simulink model "ideal_switch_inverter_one_ph_x3"  (R2025a)
settings: Solver=daessc  StartTime=0.0  StopTime=0.2  MaxStep=1e-7  RelTol=1e-3
undefined symbols (not defined in the file): Down, Up
libraries: ee_lib x33, fl_lib x19, nesl_utility x17, eePwmGenerator x6, spsMeanLib x3, simulink x2, spsRMSLib x1
settings Model: SimulationMode=rapid-accelerator  Creator=alexey  LastModifiedBy=alexey
settings SolverCC: ZeroCrossAlgorithm=Adaptive
settings OptimizationCC: ReuseModelBlockBuffer=off
settings DebuggingCC: IgnoredZcDiagnostic=none
settings RTWCC: GPUComputeCapability=3.5
settings GRTTargetCC: RTWCAPISignals=on  RTWCAPIParams=on

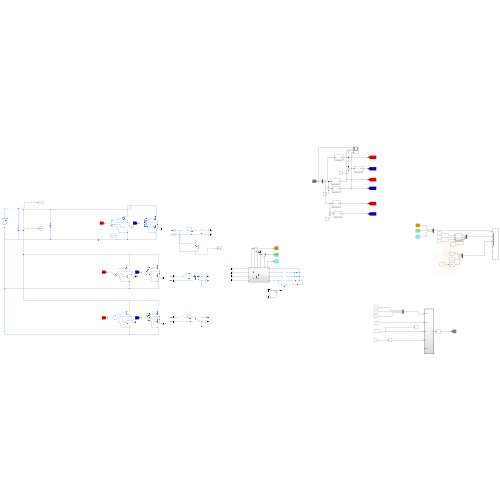
[thumbnail: Simulink's stored preview of the top-level diagram]
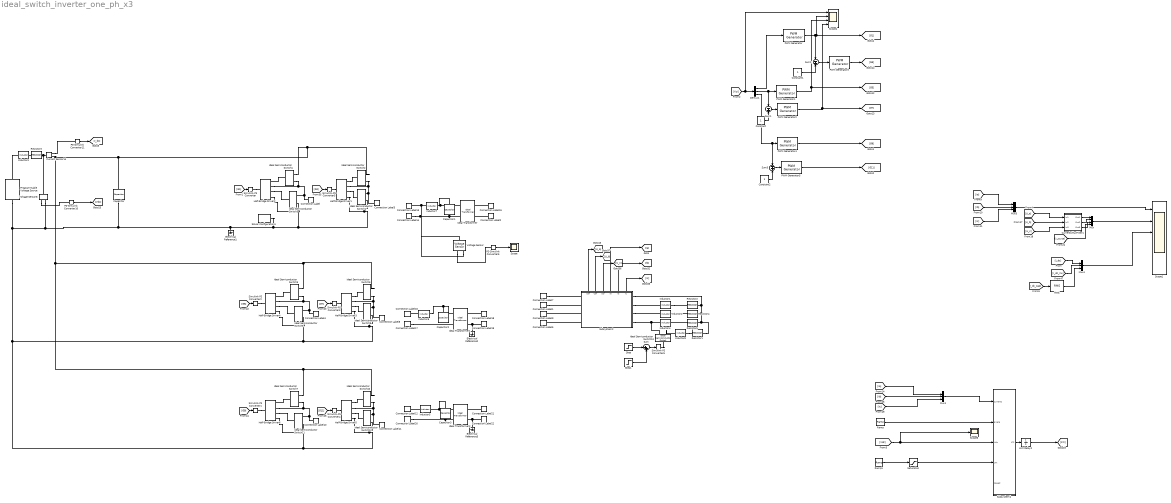
== system ideal_switch_inverter_one_ph_x3 ==
  Capacitor : fl_lib/Electrical/Electrical Elements/Capacitor  c=900 uF  r=1e-6 Ohm  g=0 1/Ohm  i_specify=off  i_priority=None  i=0 A  i_nominal_specify=off  i_nominal_value=1  i_nominal_unit=A  v_specify=off  v_priority=None  v=0 V  v_nominal_specify=off  v_nominal_value=1  v_nominal_unit=V  vc_specify=off  vc_priority=High  vc=0 V  vc_nominal_specify=off  vc_nominal_value=1  vc_nominal_unit=V
  Capacitor1 : fl_lib/Electrical/Electrical Elements/Capacitor  c=100 uF  r=2 mOhm  g=0 1/Ohm  i_specify=off  i_priority=None  i=0 A  i_nominal_specify=off  i_nominal_value=1  i_nominal_unit=A  v_specify=on  v_priority=None  v=0 V  v_nominal_specify=off  v_nominal_value=1  v_nominal_unit=V  vc_specify=off  vc_priority=High  vc=0 V  vc_nominal_specify=off  vc_nominal_value=1  vc_nominal_unit=V
  Capacitor2 : fl_lib/Electrical/Electrical Elements/Capacitor  c=100 uF  r=2 mOhm  g=0 1/Ohm  i_specify=off  i_priority=None  i=0 A  i_nominal_specify=off  i_nominal_value=1  i_nominal_unit=A  v_specify=on  v_priority=None  v=0 V  v_nominal_specify=off  v_nominal_value=1  v_nominal_unit=V  vc_specify=off  vc_priority=High  vc=0 V  vc_nominal_specify=off  vc_nominal_value=1  vc_nominal_unit=V
  Capacitor3 : fl_lib/Electrical/Electrical Elements/Capacitor  c=100 uF  r=2 mOhm  g=0 1/Ohm  i_specify=off  i_priority=None  i=0 A  i_nominal_specify=off  i_nominal_value=1  i_nominal_unit=A  v_specify=on  v_priority=None  v=0 V  v_nominal_specify=off  v_nominal_value=1  v_nominal_unit=V  vc_specify=off  vc_priority=High  vc=0 V  vc_nominal_specify=off  vc_nominal_value=1  vc_nominal_unit=V
  Connection Label : ConnectionLabel  Label=A01
  Connection Label1 : ConnectionLabel  Label=A
  Connection Label10 : ConnectionLabel  Label=C01
  Connection Label11 : ConnectionLabel  Label=C02
  Connection Label12 : ConnectionLabel  Label=C01
  Connection Label13 : ConnectionLabel  Label=A01
  Connection Label14 : ConnectionLabel  Label=A02
  Connection Label15 : ConnectionLabel  Label=A
  Connection Label16 : ConnectionLabel  Label=B01
  Connection Label17 : ConnectionLabel  Label=B02
  Connection Label18 : ConnectionLabel  Label=B
  Connection Label{2,7,19,22} (4 alike) : ConnectionLabel  Label=N
  Connection Label20 : ConnectionLabel  Label=C02
  Connection Label21 : ConnectionLabel  Label=C
  Connection Label3 : ConnectionLabel  Label=A02
  Connection Label4 : ConnectionLabel  Label=B01
  Connection Label5 : ConnectionLabel  Label=C
  Connection Label8 : ConnectionLabel  Label=B02
  Connection Label9 : ConnectionLabel  Label=B
  Constant : Constant
  Constant1 : Constant
  Constant2 : Constant
  Current Sensor14 : fl_lib/Electrical/Electrical Sensors/Current Sensor
  CurrentsMuxFilter1 : Subsystem
  Demux1 : Demux  Outputs=3
  Electrical Reference1 : fl_lib/Electrical/Electrical Elements/Electrical Reference
  Electrical Reference2 : fl_lib/Electrical/Electrical Elements/Electrical Reference
  Electrical Reference3 : fl_lib/Electrical/Electrical Elements/Electrical Reference
  Half-Bridge Driver{1..6} (6 alike) : ee_lib/Semiconductors & Converters/Half-Bridge Driver  port_option=ee.enum.controlport.ps  uHigh=2.0 V  uLow=0.8 V  uHighValue=0.7  uLowValue=0.3  vHigh=15 V  vLow=0 V  tpLH=50 ns  tdLH=1 ns  tpHL=50 ns  tdHL=1 ns  parameterization=ee.enum.semiconductors.gateDriverParam.outputImpedance  rHigh=2 Ohm  rLow=2 Ohm  tRise=20 ns  tFall=20 ns  cLoad=10 nF  ZonTime_specify=off  ZonTime_priority=None  ZonTime=0 s  ZoffTime_specify=off  ZoffTime_priority=None  ZoffTime=0 s  power_dissipated_high_side_specify=off  power_dissipated_high_side_priority=None  power_dissipated_high_side=0 W  power_dissipated_high_side_nominal_specify=off  power_dissipated_high_side_nominal_value=1  power_dissipated_high_side_nominal_unit=W  power_dissipated_low_side_specify=off  power_dissipated_low_side_priority=None  power_dissipated_low_side=0 W  power_dissipated_low_side_nominal_specify=off  power_dissipated_low_side_nominal_value=1  power_dissipated_low_side_nominal_unit=W
      settings: InternalSimscapePortConfiguration="{\"Bottom\":[],\"Left\":[{\"id\":\"u\",\"label\":\"u\",\"type\":\"input\"}],\"Right\":[{\"id\":\"HO\",\"label\":\"HO\",\"type\":\"foundation.electrical.electrical\"},{\"id\":\"HS\",\"label\":\"HS\",\"type\":\"foundation.electrical.electrical\"},{\"id\":\"LO\",\"label\":\"LO\",\"type\":\"foundation.electrical.electrical\"},{\"id\":\"LS\",\"label\":\"LS\",\"type\":\"foundation.electrical.electrical\"}],\"Top\":[]}"
  Ideal Semiconductor Switch{1..12} (12 alike) : ee_lib/Semiconductors & Converters/Ideal Semiconductor Switch  port_option=ee.enum.controlport.elec  Ron=0.001 Ohm  Goff=1e-6 1/Ohm  Vth=10 V  diode_param=ee.enum.semiconductors.protectionDiode.nodynamics  diode_Vf=0.8 V  diode_Ron=0.001 Ohm  diode_Goff=1e-5 1/Ohm  diode_C=50e-9 F  diode_iRM=-235 A  diode_iF=300 A  diode_idot=-50 A/us  diode_trr_param=ee.enum.converters.diodetrr.trr_factor  diode_trr_factor=3  diode_trr=15 us  diode_Qrr=1500 s*uA
      settings: InternalSimscapePortConfiguration="{\"Bottom\":[],\"Left\":[{\"id\":\"G_elec\",\"label\":\"\",\"type\":\"foundation.electrical.electrical\"}],\"Right\":[{\"id\":\"A\",\"label\":\"a\",\"type\":\"foundation.electrical.electrical\"},{\"id\":\"K\",\"label\":\"k\",\"type\":\"foundation.electrical.electrical\"}],\"Top\":[]}"
  Ideal Semiconductor Switch13 : ee_lib/Semiconductors & Converters/Ideal Semiconductor Switch  port_option=ee.enum.controlport.ps  Ron=0.001 Ohm  Goff=1e-6 1/Ohm  Vth=1.5 V  diode_param=ee.enum.semiconductors.protectionDiode.external  diode_Vf=0.8 V  diode_Ron=0.001 Ohm  diode_Goff=1e-5 1/Ohm  diode_C=50e-9 F  diode_iRM=-235 A  diode_iF=300 A  diode_idot=-50 A/us  diode_trr_param=ee.enum.converters.diodetrr.trr_factor  diode_trr_factor=3  diode_trr=15 us  diode_Qrr=1500 s*uA
  Ideal Transformer : fl_lib/Electrical/Electrical Elements/Ideal Transformer  n=1  i1_specify=off  i1_priority=None  i1=0 A  i1_nominal_specify=off  i1_nominal_value=1  i1_nominal_unit=A  v1_specify=off  v1_priority=None  v1=0 V  v1_nominal_specify=off  v1_nominal_value=1  v1_nominal_unit=V  i2_specify=off  i2_priority=None  i2=0 A  i2_nominal_specify=off  i2_nominal_value=1  i2_nominal_unit=A  v2_specify=off  v2_priority=None  v2=0 V  v2_nominal_specify=off  v2_nominal_value=1  v2_nominal_unit=V
  Ideal Transformer1 : fl_lib/Electrical/Electrical Elements/Ideal Transformer  n=1  i1_specify=off  i1_priority=None  i1=0 A  i1_nominal_specify=off  i1_nominal_value=1  i1_nominal_unit=A  v1_specify=off  v1_priority=None  v1=0 V  v1_nominal_specify=off  v1_nominal_value=1  v1_nominal_unit=V  i2_specify=off  i2_priority=None  i2=0 A  i2_nominal_specify=off  i2_nominal_value=1  i2_nominal_unit=A  v2_specify=off  v2_priority=None  v2=0 V  v2_nominal_specify=off  v2_nominal_value=1  v2_nominal_unit=V
  Ideal Transformer2 : fl_lib/Electrical/Electrical Elements/Ideal Transformer  n=1  i1_specify=off  i1_priority=None  i1=0 A  i1_nominal_specify=off  i1_nominal_value=1  i1_nominal_unit=A  v1_specify=off  v1_priority=None  v1=0 V  v1_nominal_specify=off  v1_nominal_value=1  v1_nominal_unit=V  i2_specify=off  i2_priority=None  i2=0 A  i2_nominal_specify=off  i2_nominal_value=1  i2_nominal_unit=A  v2_specify=off  v2_priority=None  v2=0 V  v2_nominal_specify=off  v2_nominal_value=1  v2_nominal_unit=V
  Inductor{1..2,4,8} (4 alike) : ee_lib/Passive/Inductor  l=3630 uH  enable_L_tol=0  L_tol=20  tol_distribution=1  nSigma=4  r=0 Ohm  g=1e-9 1/Ohm  enable_operating_limits=0  operating_limit_action=2  max_working_current=1 A  power_rating=1 W  i_L_specify=on  i_L_priority=High  i_L=0 A  i_L_nominal_specify=off  i_L_nominal_value=1  i_L_nominal_unit=A
  Inductor3 : ee_lib/Passive/Inductor  l=1 uH  enable_L_tol=0  L_tol=20  tol_distribution=1  nSigma=4  r=0 Ohm  g=1e-9 1/Ohm  enable_operating_limits=0  operating_limit_action=2  max_working_current=1 A  power_rating=1 W  i_L_specify=on  i_L_priority=High  i_L=0 A  i_L_nominal_specify=off  i_L_nominal_value=1  i_L_nominal_unit=A
  Inductor5 : ee_lib/Passive/Inductor  l=200 uH  enable_L_tol=0  L_tol=20  tol_distribution=1  nSigma=4  r=0 Ohm  g=1e-9 1/Ohm  enable_operating_limits=0  operating_limit_action=2  max_working_current=1 A  power_rating=1 W  i_L_specify=on  i_L_priority=High  i_L=0 A  i_L_nominal_specify=off  i_L_nominal_value=1  i_L_nominal_unit=A
  Inductor6 : ee_lib/Passive/Inductor  l=200 uH  enable_L_tol=0  L_tol=20  tol_distribution=1  nSigma=4  r=0 Ohm  g=1e-9 1/Ohm  enable_operating_limits=0  operating_limit_action=2  max_working_current=1 A  power_rating=1 W  i_L_specify=on  i_L_priority=High  i_L=0 A  i_L_nominal_specify=off  i_L_nominal_value=1  i_L_nominal_unit=A
  Inductor7 : ee_lib/Passive/Inductor  l=200 uH  enable_L_tol=0  L_tol=20  tol_distribution=1  nSigma=4  r=0 Ohm  g=1e-9 1/Ohm  enable_operating_limits=0  operating_limit_action=2  max_working_current=1 A  power_rating=1 W  i_L_specify=on  i_L_priority=High  i_L=0 A  i_L_nominal_specify=off  i_L_nominal_value=1  i_L_nominal_unit=A
  Mux : Mux
  Mux1 : Mux  Inputs=3
  Mux3 : Mux  Inputs=3
  Mux4 : Mux  Inputs=3
  PS-Simulink Converter10 : nesl_utility/PS-Simulink Converter  PhysicalDomain=network_engine_domain  SubClassName=ps_output  LeftPortType=input  RightPortType=output  PseudoPeriodic=off  Frequencies=[]  VectorFormat=inherit  Unit=inherit  AffineConversion=off
  PS-Simulink Converter11 : nesl_utility/PS-Simulink Converter  PhysicalDomain=network_engine_domain  SubClassName=ps_output  LeftPortType=input  RightPortType=output  PseudoPeriodic=off  Frequencies=[]  VectorFormat=inherit  Unit=inherit  AffineConversion=off
  PS-Simulink Converter5 : nesl_utility/PS-Simulink Converter  PhysicalDomain=network_engine_domain  SubClassName=ps_output  LeftPortType=input  RightPortType=output  PseudoPeriodic=off  Frequencies=[]  VectorFormat=inherit  Unit=inherit  AffineConversion=off
  PWM Generator{,1..5} (6 alike) : eePwmGenerator/PWM Generator  CarrCount=Up-Down  Tper=0.5/10000  Tdelay=0  Ts=100e-9
  Programmable Voltage Source : ee_lib/Sources/Programmable Voltage Source  magnitude_type=ee.enum.timechanging.constant  ac_magnitude=0 V  magn_ramp=1 V/s  magn_step=1 V  magn_modu_magn=1 V  magn_modu_freq=1 Hz  magn_t1=1 s  magn_t2=2 s  frequency_type=ee.enum.timechanging.constant  ac_frequency=60 Hz  freq_ramp=1 Hz/s  freq_step=1 Hz  freq_modu_magn=1 Hz  freq_modu_freq=1 Hz  freq_t1=1 s  freq_t2=2 s  phase_type=ee.enum.timechanging.constant  ac_shift=0 deg  phase_ramp=1 deg/s  phase_step=1 deg  phase_modu_magn=1 deg  phase_modu_freq=1 Hz  phase_t1=1 s  phase_t2=2 s  dc_type=ee.enum.timechanging.ramp  dc_voltage=0 V  dc_ramp=450000 V/s  dc_step=24 V  dc_modu_magn=1 V  dc_modu_freq=1 Hz  dc_t1=0 s  dc_t2=100e-5 s  harmonic_option=0  harmonic_orders=[5, 7, 11, 13]  harmonic_ratios=[.1, .1, .1, .1]  harmonic_shifts=[0, 0, 0, 0] deg  harmonic_t1=-inf s  harmonic_t2=inf s  noise_mode=0  PSD=0 V^2/Hz  repeatability=1  auto_seed=0  user_seed=0  sample_time=1e-3 s  i_specify=off  i_priority=None  i=0 A  i_nominal_specify=off  i_nominal_value=1  i_nominal_unit=A  v_specify=on  v_priority=High  v=0 V  v_nominal_specify=off  v_nominal_value=1  v_nominal_unit=V
      settings: InternalSimscapePortConfiguration="{\"Bottom\":[],\"Left\":[{\"id\":\"p\",\"label\":\"+\",\"type\":\"foundation.electrical.electrical\"}],\"Right\":[{\"id\":\"n\",\"label\":\"-\",\"type\":\"foundation.electrical.electrical\"}],\"Top\":[]}"
  RMS : spsRMSLib/RMS  TrueRMS=on  Freq=1000  RMSInit=0  Ts=0
  Ramp : simulink/Sources/Ramp  slope=100*pi  start=0  InitialOutput=0
  Ramp1 : simulink/Sources/Ramp  slope=7500  start=0  InitialOutput=0
  Resistor1 : ee_lib/Passive/Resistor  R=1.52 Ohm  enable_R_tol=0  R_tol=5  tol_distribution=1  nSigma=4  enable_operating_limits=0  operating_limit_action=2  power_rating=1 W  max_working_voltage=100 V  noise_mode=0  Tdevice=25 degC  sample_time=1e-3 s  repeatability=1  user_seed=0  auto_seed=1003532619  power_derating_T1=70 degC  power_derating_T2=155 degC  operating_temperature_range_vec=[-50, 150] degC  alpha=3.93e-3 1/K  Tmeas=25 degC  thermal_mass=100 J/K  temperature_specify=off  temperature_priority=High  temperature=298.15 K  temperature_nominal_specify=off  temperature_nominal_value=1  temperature_nominal_unit=K
  Resistor2 : ee_lib/Passive/Resistor  R=1.52 Ohm  enable_R_tol=0  R_tol=5  tol_distribution=1  nSigma=4  enable_operating_limits=0  operating_limit_action=2  power_rating=1 W  max_working_voltage=100 V  noise_mode=0  Tdevice=25 degC  sample_time=1e-3 s  repeatability=1  user_seed=0  auto_seed=1045931777  power_derating_T1=70 degC  power_derating_T2=155 degC  operating_temperature_range_vec=[-50, 150] degC  alpha=3.93e-3 1/K  Tmeas=25 degC  thermal_mass=100 J/K  temperature_specify=off  temperature_priority=High  temperature=298.15 K  temperature_nominal_specify=off  temperature_nominal_value=1  temperature_nominal_unit=K
  Resistor3 : ee_lib/Passive/Resistor  R=1 mOhm  enable_R_tol=0  R_tol=5  tol_distribution=1  nSigma=4  enable_operating_limits=0  operating_limit_action=2  power_rating=1 W  max_working_voltage=100 V  noise_mode=0  Tdevice=25 degC  sample_time=1e-3 s  repeatability=1  user_seed=0  auto_seed=545404223  power_derating_T1=70 degC  power_derating_T2=155 degC  operating_temperature_range_vec=[-50, 150] degC  alpha=3.93e-3 1/K  Tmeas=25 degC  thermal_mass=100 J/K  temperature_specify=off  temperature_priority=High  temperature=298.15 K  temperature_nominal_specify=off  temperature_nominal_value=1  temperature_nominal_unit=K
  Resistor4 : ee_lib/Passive/Resistor  R=1.52 Ohm  enable_R_tol=0  R_tol=5  tol_distribution=1  nSigma=4  enable_operating_limits=0  operating_limit_action=2  power_rating=1 W  max_working_voltage=100 V  noise_mode=0  Tdevice=25 degC  sample_time=1e-3 s  repeatability=1  user_seed=0  auto_seed=844370171  power_derating_T1=70 degC  power_derating_T2=155 degC  operating_temperature_range_vec=[-50, 150] degC  alpha=3.93e-3 1/K  Tmeas=25 degC  thermal_mass=100 J/K  temperature_specify=off  temperature_priority=High  temperature=298.15 K  temperature_nominal_specify=off  temperature_nominal_value=1  temperature_nominal_unit=K
  Resistor5 : ee_lib/Passive/Resistor  R=1.52 Ohm  enable_R_tol=0  R_tol=5  tol_distribution=1  nSigma=4  enable_operating_limits=0  operating_limit_action=2  power_rating=1 W  max_working_voltage=100 V  noise_mode=0  Tdevice=25 degC  sample_time=1e-3 s  repeatability=1  user_seed=0  auto_seed=1078396959  power_derating_T1=70 degC  power_derating_T2=155 degC  operating_temperature_range_vec=[-50, 150] degC  alpha=3.93e-3 1/K  Tmeas=25 degC  thermal_mass=100 J/K  temperature_specify=off  temperature_priority=High  temperature=298.15 K  temperature_nominal_specify=off  temperature_nominal_value=1  temperature_nominal_unit=K
  Saturation : Saturate  UpperLimit=450
  Scope : Scope
      settings: ActiveDisplayYMinimum=-551.33280842234649  ActiveDisplayYMaximum=616.82988904528236
  Scope1 : Scope  NumInputPorts=6
      settings: ActiveDisplayString=6  ActiveDisplayYMinimum=-1  ActiveDisplayYMaximum=1
  Scope4 : Scope  NumInputPorts=4
      settings: ActiveDisplayYMinimum=-0.081880277547520586  ActiveDisplayYMaximum=0.73692249792768538  DataLoggingVariableName=ScopeData2
  Scope6 : Scope
      settings: ActiveDisplayYMinimum=-58.427844353684108  ActiveDisplayYMaximum=525.8505991831571  DataLoggingVariableName=ScopeData4
  Simulink-PS Converter{,1..6} (7 alike) : nesl_utility/Simulink-PS Converter  PhysicalDomain=network_engine_domain  SubClassName=ps_input  LeftPortType=input  RightPortType=output  PseudoPeriodic=off  Frequencies=[]  NoiseDistribution=none  NoiseParameters=[]  Unit=1  AffineConversion=off  FilteringAndDerivatives=provide  SimscapeFilterOrder=1  InputFilterTimeConstant=0.001  UdotUserProvided=0
  Solver Configuration1 : nesl_utility/Solver Configuration  PhysicalDomain=network_engine_domain  SubClassName=solver  LeftPortType=input  RightPortType=generic  Tones=[]  Harmonics=[]  SimulateNoise=off  Profile=off  UseLocalSampling=off  EnableSwitchedLinearOptims=on  FrequencyDomain=off  UseCCode=off  RelTol=0.001  AbsTol=0.001  MinStep=1e-09  ToWorkspace=off  RevertToSquareIcSolve=off  NumHomotopyIterations=100  PhasorMode=off  PhasorModeNumHarmonics=1  ConsistencySolver=NEWTON_XTOL_AFTER_FTOL  IndexReductionMethod=DerivativeReplacement  DoDC=off  ResidualTolerance=1e-09  ConsistencyTolSource=GLOBAL  ConsistencyAbsTol=0.001  ConsistencyRelTol=0.001  ConsistencyTolFactor=0.001  UseLocalSolver=off  LocalSolverChoice=NE_BACKWARD_EULER_ADVANCER  ResolveIndetEquations=on  FunctionEvalNumThread=1  LocalSolverSampleTime=0.001  DoFixedCost=off  MaxNonlinIter=3  MaxModeIter=2  ComputeImpulses=off  ImpulseIterations=2  LinearAlgebra=auto  LinearAlgebraNumThread=0  EquationFormulation=NE_TIME_EF  DelaysMemoryBudget=1024  AutomaticFiltering=on  FilteringTimeConstant=0.001  PartitionStorageMethod=AS_NEEDED  PartitionMemoryBudget=1024  PartitionMethod=ROBUST  MultibodyUseLocalSolver=off  MultibodyLocalSolverChoice=ODE1  MultibodyLocalSolverSampleTime=0.001
  Step : Step  Time=0.08  SampleTime=0
  Step1 : Step  Time=0.12  Before=1  After=0  SampleTime=0
  Subsystem1 : Subsystem  TreatAsAtomicUnit=on  SystemSampleTime=1/10000
  Subsystem2 : Subsystem
      settings: PortSchema="{\"entries\":[{\"content\":{\"sides\":[{\"content\":{},\"type\":\"ConnectorPlacement.EquallySpacedRectSide\",\"uuid\":\"18ff9a98-da5f-4d42-bf88-8b80acaefaab\"},{\"content\":{\"connectorIds\":[\"Out1\",\"Out2\",\"Out3\",\"Out4\",\"Out5\",\"Out6\"],\"side\":\"RIGHT\"},\"type\":\"ConnectorPlacement.EquallySpacedRectSide\",\"uuid\":\"2ae2e449-c022-4e43-8d74-e7903f555369\"},{\"content\":{\"connectorIds\":[\"LConn1\",\"LConn2\",\"LConn3\",\"LConn4\"],\"side\":\"TOP\"},\"type\":\"ConnectorPlacement.EquallySpacedRectSide\",\"uuid\":\"55b123c9-903d-428f-ba92-02a5913ccae5\"},{\"content\":{\"connectorIds\":[\"RConn1\",\"RConn2\",\"RConn3\",\"RConn4\"],\"side\":\"BOTTOM\"},\"type\":\"ConnectorPlacement.EquallySpacedRectSide\",\"uuid\":\"b028b0af-4fd3-4535-8d3b-f50dc0cabb29\"}]},\"type\":\"ConnectorPlacement.EquallySpacedConnector\",\"uuid\":\"08d0fd08-360e-4301-974e-a78b2c2bf0b9\"}],\"packageUris\":[\"http://schema.mathworks.com/mf0/Connector/R2020b\"],\"version\":\"1.0\"}"
  Sum : Sum  Inputs=|++
  Sum1 : Sum  Inputs=-+
  Sum2 : Sum  Inputs=-+
  Sum3 : Sum  Inputs=-+
  Unit Delay2 : UnitDelay  SampleTime=-1  HasFrameUpgradeWarning=on
  Voltage Sensor : fl_lib/Electrical/Electrical Sensors/Voltage Sensor
  Voltage Sensor8 : fl_lib/Electrical/Electrical Sensors/Voltage Sensor
  wires:
  [Ib] -> Mux1/2
  [Ia] -> Mux1/1
  PS-Simulink Converter10/1 -> [Vdc]
  [G1] -> Simulink-PS Converter/1
  PS-Simulink Converter11/1 -> [I_dc]
  [G3] -> Simulink-PS Converter5/1
  [Vdc] -> Scope6/1, Subsystem1/3(Vdc)
  [I_dc] -> Mux4/1
  Subsystem1/1(KZI) -> Unit Delay2/1
  Unit Delay2/1 -> [Kzi]
  [Kzi] -> Scope4/1, Demux1/1
  Demux1/1 -> PWM Generator/1
  Demux1/2 -> PWM Generator1/1, Sum1/1
  PWM Generator1/1 -> Scope4/3, [G5]
  PWM Generator2/1 -> [G7], Scope4/4
  [I_dc_inv] -> Mux4/2
  [Ia] -> Mux3/1
  [Ib] -> Mux3/2
  [Ic] -> Mux3/3
  Mux4/1 -> Scope1/3
  Subsystem2/1(Uaf) -> [U_a]
  Subsystem2/2(Ubf) -> [U_b]
  Subsystem2/3(Ucf) -> [U_c]
  Subsystem2/4(Ia) -> [Ia]
  Subsystem2/5(Ib) -> [Ib]
  Subsystem2/6(Ic) -> [Ic]
  [U_a] -> CurrentsMuxFilter1/1(In1)
  [U_b] -> CurrentsMuxFilter1/2(In2)
  [U_c] -> CurrentsMuxFilter1/3(In3)
  CurrentsMuxFilter1/1(Out1) -> Mux/1
  CurrentsMuxFilter1/2(Out2) -> Mux/2
  CurrentsMuxFilter1/3(Out3) -> Mux/3
  Mux/1 -> Scope1/2
  Mux3/1 -> Scope1/1
  [Ic] -> Mux1/3
  Mux1/1 -> Subsystem1/1(currents)
  [v_source] -> Mux/4
  [I_dc_cap] -> RMS/1
  Ramp/1 -> Subsystem1/2(angle)
  RMS/1 -> Mux4/3
  Ramp1/1 -> Saturation/1
  Saturation/1 -> Subsystem1/4(Um)
  Constant/1 -> Sum1/2
  Sum1/1 -> PWM Generator2/1
  Sum2/1 -> PWM Generator3/1
  Constant1/1 -> Sum2/2
  PWM Generator/1 -> Scope4/2, [G1], Sum2/1
  PWM Generator3/1 -> [G3]
  [G7] -> Simulink-PS Converter3/1
  [G5] -> Simulink-PS Converter2/1
  [G9] -> Simulink-PS Converter1/1
  [G11] -> Simulink-PS Converter4/1
  Sum3/1 -> PWM Generator5/1
  Constant2/1 -> Sum3/2
  PWM Generator5/1 -> [G11]
  Demux1/3 -> Sum3/1, PWM Generator4/1
  PWM Generator4/1 -> [G9]
  Step/1 -> Sum/1
  Step1/1 -> Sum/2
  PS-Simulink Converter5/1 -> Scope/1
  Sum/1 -> Simulink-PS Converter6/1
  connections:
  Resistor3/RConn1 -- Inductor3/RConn1
  Ideal Semiconductor Switch1/LConn1 -- Half-Bridge Driver2/RConn1
  Inductor3/LConn1 -- Programmable Voltage Source/LConn1
  Half-Bridge Driver1/RConn1 -- Ideal Semiconductor Switch2/LConn1
  Current Sensor14/LConn1 -- Voltage Sensor8/LConn1 -- Resistor3/LConn1
  Half-Bridge Driver2/RConn3 -- Ideal Semiconductor Switch3/LConn1
  Voltage Sensor8/RConn1 -- PS-Simulink Converter10/LConn1
  Simulink-PS Converter5/RConn1 -- Half-Bridge Driver1/LConn1
  Simulink-PS Converter/RConn1 -- Half-Bridge Driver2/LConn1
  Current Sensor14/RConn1 -- PS-Simulink Converter11/LConn1
  Half-Bridge Driver1/RConn3 -- Ideal Semiconductor Switch4/LConn1
  Half-Bridge Driver6/RConn4 -- Half-Bridge Driver1/RConn4 -- Ideal Semiconductor Switch4/RConn2 -- Half-Bridge Driver2/RConn4 -- Ideal Semiconductor Switch3/RConn2 -- Solver Configuration1/RConn1 -- Electrical Reference1/LConn1 -- Capacitor/RConn1 -- Voltage Sensor8/RConn2 -- Programmable Voltage Source/RConn1 -- Half-Bridge Driver4/RConn4 -- Ideal Semiconductor Switch8/RConn2 -- Ideal Semiconductor Switch9/RConn2 -- Half-Bridge Driver3/RConn4 -- Half-Bridge Driver5/RConn4 -- Ideal Semiconductor Switch12/RConn2 -- Ideal Semiconductor Switch11/RConn2
  Half-Bridge Driver1/RConn2 -- Connection Label3/LConn1 -- Ideal Semiconductor Switch4/RConn1 -- Ideal Semiconductor Switch2/RConn2
  Half-Bridge Driver2/RConn2 -- Ideal Semiconductor Switch1/RConn2 -- Connection Label/LConn1 -- Ideal Semiconductor Switch3/RConn1
  Connection Label1/LConn1 -- Subsystem2/LConn3
  Subsystem2/LConn2 -- Connection Label9/LConn1
  Subsystem2/LConn1 -- Connection Label5/LConn1
  Inductor1/RConn1 -- Resistor2/RConn1
  Resistor4/RConn1 -- Inductor2/RConn1
  Resistor5/RConn1 -- Inductor4/RConn1
  Resistor2/LConn1 -- Subsystem2/RConn4 -- Resistor1/LConn1 -- Resistor5/LConn1 -- Resistor4/LConn1
  Subsystem2/RConn3 -- Inductor1/LConn1
  Subsystem2/RConn2 -- Inductor2/LConn1
  Subsystem2/RConn1 -- Inductor4/LConn1 -- Ideal Semiconductor Switch13/RConn1
  Connection Label7/LConn1 -- Subsystem2/LConn4
  Connection Label14/LConn1 -- Voltage Sensor/RConn2 -- Capacitor1/RConn1 -- Ideal Transformer/LConn2
  Ideal Transformer/LConn1 -- Capacitor1/LConn1 -- Inductor7/RConn1
  Connection Label2/LConn1 -- Ideal Transformer/RConn2
  Connection Label15/LConn1 -- Ideal Transformer/RConn1
  Connection Label17/LConn1 -- Ideal Transformer1/LConn2
  Inductor6/RConn1 -- Capacitor2/LConn1 -- Ideal Transformer1/LConn1
  Connection Label18/LConn1 -- Ideal Transformer1/RConn1
  Connection Label19/LConn1 -- Electrical Reference2/LConn1 -- Ideal Transformer1/RConn2
  Half-Bridge Driver3/RConn2 -- Ideal Semiconductor Switch6/RConn2 -- Ideal Semiconductor Switch9/RConn1 -- Connection Label8/LConn1
  Half-Bridge Driver4/RConn2 -- Ideal Semiconductor Switch8/RConn1 -- Connection Label4/LConn1 -- Ideal Semiconductor Switch5/RConn2
  Ideal Semiconductor Switch7/RConn1 -- Ideal Semiconductor Switch5/RConn1 -- Ideal Semiconductor Switch6/RConn1 -- Current Sensor14/RConn2 -- Capacitor/LConn1 -- Ideal Semiconductor Switch1/RConn1 -- Ideal Semiconductor Switch2/RConn1 -- Ideal Semiconductor Switch10/RConn1
  Half-Bridge Driver3/RConn3 -- Ideal Semiconductor Switch9/LConn1
  Simulink-PS Converter2/RConn1 -- Half-Bridge Driver4/LConn1
  Simulink-PS Converter3/RConn1 -- Half-Bridge Driver3/LConn1
  Half-Bridge Driver4/RConn3 -- Ideal Semiconductor Switch8/LConn1
  Half-Bridge Driver3/RConn1 -- Ideal Semiconductor Switch6/LConn1
  Ideal Semiconductor Switch5/LConn1 -- Half-Bridge Driver4/RConn1
  Inductor7/LConn1 -- Voltage Sensor/LConn1 -- Connection Label13/LConn1
  Inductor6/LConn1 -- Connection Label16/LConn1
  Ideal Semiconductor Switch12/RConn1 -- Half-Bridge Driver5/RConn2 -- Ideal Semiconductor Switch10/RConn2 -- Connection Label11/LConn1
  Ideal Semiconductor Switch11/RConn1 -- Half-Bridge Driver6/RConn2 -- Ideal Semiconductor Switch7/RConn2 -- Connection Label10/LConn1
  Simulink-PS Converter1/RConn1 -- Half-Bridge Driver6/LConn1
  Ideal Semiconductor Switch7/LConn1 -- Half-Bridge Driver6/RConn1
  Half-Bridge Driver5/RConn1 -- Ideal Semiconductor Switch10/LConn1
  Half-Bridge Driver5/RConn3 -- Ideal Semiconductor Switch12/LConn1
  Simulink-PS Converter4/RConn1 -- Half-Bridge Driver5/LConn1
  Half-Bridge Driver6/RConn3 -- Ideal Semiconductor Switch11/LConn1
  Connection Label20/LConn1 -- Capacitor3/RConn1 -- Ideal Transformer2/LConn2
  Ideal Transformer2/LConn1 -- Capacitor3/LConn1 -- Inductor5/RConn1
  Electrical Reference3/LConn1 -- Connection Label22/LConn1 -- Ideal Transformer2/RConn2
  Connection Label21/LConn1 -- Ideal Transformer2/RConn1
  Inductor5/LConn1 -- Connection Label12/LConn1
  Voltage Sensor/RConn1 -- PS-Simulink Converter5/LConn1
  Simulink-PS Converter6/RConn1 -- Ideal Semiconductor Switch13/LConn1
  Inductor8/RConn1 -- Resistor1/RConn1
  Ideal Semiconductor Switch13/RConn2 -- Inductor8/LConn1

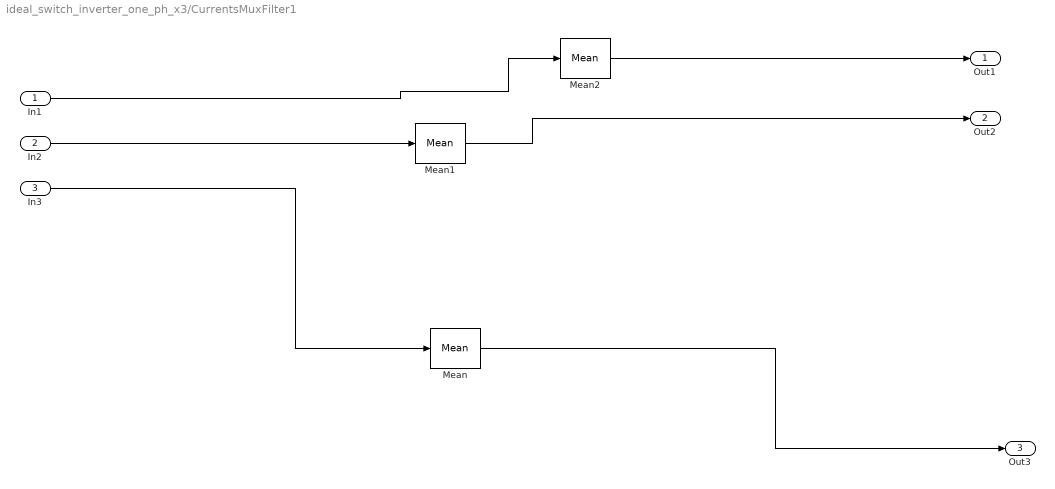
== system ideal_switch_inverter_one_ph_x3/CurrentsMuxFilter1 ==
  In1 : Inport
  In2 : Inport  Port=2
  In3 : Inport  Port=3
  Mean : spsMeanLib/Mean  Freq=10000  Vinit=0  Ts=0
  Mean1 : spsMeanLib/Mean  Freq=10000  Vinit=0  Ts=0
  Mean2 : spsMeanLib/Mean  Freq=10000  Vinit=0  Ts=0
  Out1 : Outport
  Out2 : Outport  Port=2
  Out3 : Outport  Port=3
  wires:
  In1/1 -> Mean2/1
  In3/1 -> Mean/1
  In2/1 -> Mean1/1
  Mean/1 -> Out3/1
  Mean1/1 -> Out2/1
  Mean2/1 -> Out1/1

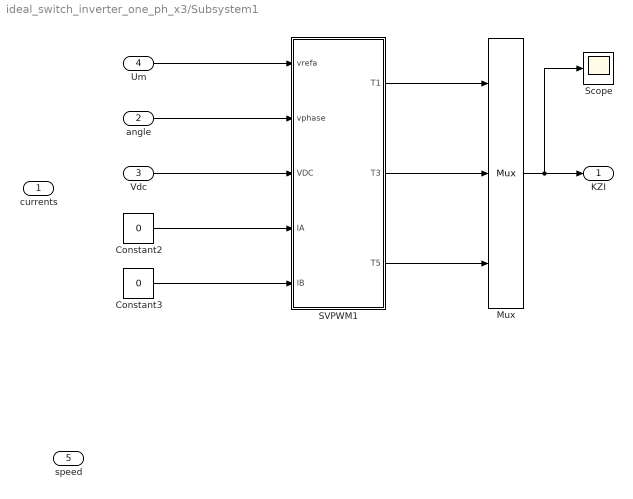
== system ideal_switch_inverter_one_ph_x3/Subsystem1 ==
  currents : Inport
  angle : Inport  Port=2
  Vdc : Inport  Port=3
  Um : Inport  Port=4
  speed : Inport  Port=5
  Constant2 : Constant  Value=0
  Constant3 : Constant  Value=0
  Mux : Mux  Inputs=3
  SVPWM1 : MATLAB Function  TreatAsAtomicUnit=on
  Scope : Scope
      settings: ActiveDisplayYMinimum=0.18750000000000003  ActiveDisplayYMaximum=0.8125  DataLoggingVariableName=ScopeData3
  KZI : Outport
  wires:
  SVPWM1/1(T1) -> Mux/1
  SVPWM1/2(T3) -> Mux/2
  SVPWM1/3(T5) -> Mux/3
  Mux/1 -> Scope/1, KZI/1
  Um/1 -> SVPWM1/1(vrefa)
  Vdc/1 -> SVPWM1/3(VDC)
  angle/1 -> SVPWM1/2(vphase)
  Constant2/1 -> SVPWM1/4(IA)
  Constant3/1 -> SVPWM1/5(IB)

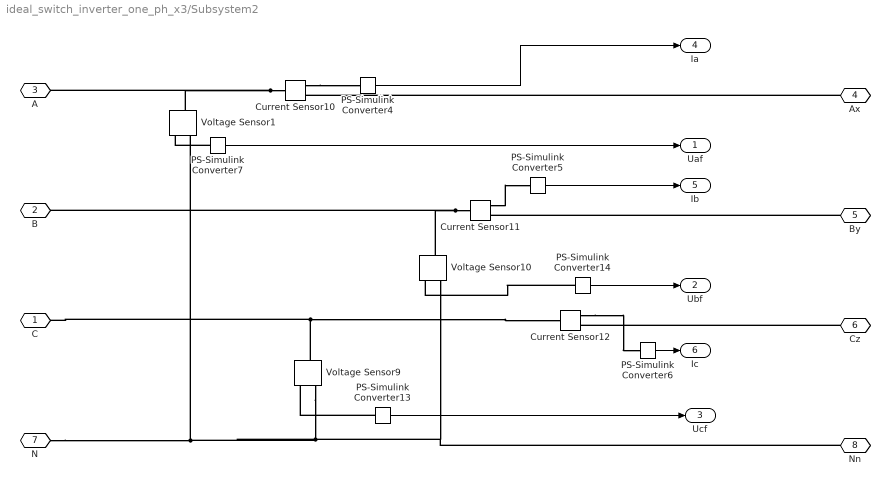
== system ideal_switch_inverter_one_ph_x3/Subsystem2 ==
  Current Sensor10 : fl_lib/Electrical/Electrical Sensors/Current Sensor
  Current Sensor11 : fl_lib/Electrical/Electrical Sensors/Current Sensor
  Current Sensor12 : fl_lib/Electrical/Electrical Sensors/Current Sensor
  PS-Simulink Converter{4..7,13..14} (6 alike) : nesl_utility/PS-Simulink Converter  PhysicalDomain=network_engine_domain  SubClassName=ps_output  LeftPortType=input  RightPortType=output  PseudoPeriodic=off  Frequencies=[]  VectorFormat=inherit  Unit=inherit  AffineConversion=off
  Voltage Sensor1 : fl_lib/Electrical/Electrical Sensors/Voltage Sensor
  Voltage Sensor10 : fl_lib/Electrical/Electrical Sensors/Voltage Sensor
  Voltage Sensor9 : fl_lib/Electrical/Electrical Sensors/Voltage Sensor
  C : PMIOPort  Side=Left
  B : PMIOPort  Port=2  Side=Left
  A : PMIOPort  Port=3  Side=Left
  Ax : PMIOPort  Port=4  Side=Right
  By : PMIOPort  Port=5  Side=Right
  Cz : PMIOPort  Port=6  Side=Right
  N : PMIOPort  Port=7  Side=Left
  Nn : PMIOPort  Port=8  Side=Right
  Uaf : Outport
  Ubf : Outport  Port=2
  Ucf : Outport  Port=3
  Ia : Outport  Port=4
  Ib : Outport  Port=5
  Ic : Outport  Port=6
  wires:
  PS-Simulink Converter7/1 -> Uaf/1
  PS-Simulink Converter14/1 -> Ubf/1
  PS-Simulink Converter4/1 -> Ia/1
  PS-Simulink Converter13/1 -> Ucf/1
  PS-Simulink Converter6/1 -> Ic/1
  PS-Simulink Converter5/1 -> Ib/1
  connections:
  By/RConn1 -- Current Sensor11/RConn2
  PS-Simulink Converter7/LConn1 -- Voltage Sensor1/RConn1
  PS-Simulink Converter14/LConn1 -- Voltage Sensor10/RConn1
  Current Sensor11/LConn1 -- B/RConn1 -- Voltage Sensor10/LConn1
  Current Sensor12/RConn1 -- PS-Simulink Converter6/LConn1
  Current Sensor10/LConn1 -- A/RConn1 -- Voltage Sensor1/LConn1
  Voltage Sensor9/LConn1 -- C/RConn1 -- Current Sensor12/LConn1
  Current Sensor11/RConn1 -- PS-Simulink Converter5/LConn1
  Cz/RConn1 -- Current Sensor12/RConn2
  Current Sensor10/RConn1 -- PS-Simulink Converter4/LConn1
  PS-Simulink Converter13/LConn1 -- Voltage Sensor9/RConn1
  Ax/RConn1 -- Current Sensor10/RConn2
  N/RConn1 -- Voltage Sensor1/RConn2 -- Voltage Sensor9/RConn2 -- Voltage Sensor10/RConn2 -- Nn/RConn1

== matlab function ideal_switch_inverter_one_ph_x3/Subsystem1/SVPWM1 ==
  data: vrefa input; vphase input; VDC input; IA input; IB input; T1 output; T3 output; T5 output
function [T1, T3, T5] = fcn(vrefa,vphase,VDC,IA,IB)
%function Ts   = fcn(vrefa,vphase,VDC,IA,IB)
%время ШИМ периода
dt=1/10000;
compensate = 0;

%алгоритм формирования векторной ШИМ  мертвым веменем dead [мкс]
dead=0.0; % in us
dead_time=dead/(dt*1e6);

phaseA = sin(vphase);
phaseB = sin(vphase - 2*pi/3);
phaseC = sin(vphase - 4*pi/3);

T1 = 0.5 + 0.5 * vrefa * phaseA / VDC;
T3 = 0.5 + 0.5 * vrefa * phaseB / VDC;
T5 = 0.5 + 0.5 * vrefa * phaseC / VDC;







if compensate == 1
    if (IA > 0) 
        T1 = T1 - dead_time/2;
        
    else
        T1 = T1 + dead_time/2;
         
    end

    if (IB > 0) 
        T3 = T3 - dead_time/2;

    else
        T3 = T3 + dead_time/2;

    end

    if (-(IA+IB) > 0) 
        T5 = T5 - dead_time/2;

    else
        T5 = T5 + dead_time/2;
          
    end
end


return;
